simulink model "HW1"  (R2017a)
settings: Solver=VariableStepAuto  StartTime=0.0  StopTime=10.0  RelTol=1e-3
settings Model: Creator=rahul  LastModifiedBy=rahul

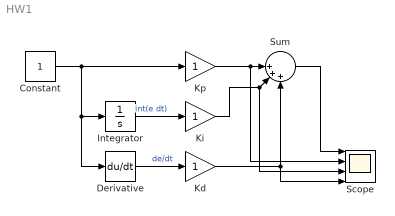
== system HW1 ==
  Constant : Constant
  Derivative : Derivative
  Integrator : Integrator
  Kd : Gain
  Ki : Gain
  Kp : Gain
  Scope : Scope  NumInputPorts=4
  Sum : Sum  Inputs=||+++
  wires:
  Integrator/1 -> Ki/1  "int(e dt)"
  Derivative/1 -> Kd/1  "de/dt"
  Constant/1 -> Kp/1, Derivative/1, Integrator/1
  Kp/1 -> Scope/2, Sum/1
  Ki/1 -> Scope/3, Sum/2
  Kd/1 -> Scope/4, Sum/3
  Sum/1 -> Scope/1
